simulink model "ieee_6_bus_modified"  (R2015b)
settings: Solver=VariableStepAuto  StartTime=0.0  StopTime=25  RelTol=1e-3
values from neighbouring files (symbols this model uses):
  Cbase = 1/(100*pi*Xbase)    (= 1.34217357979e-05)    [ieee_6_bus.m]
  Lbase = Xbase/(100*pi)    (= 0.754903726073)    [ieee_6_bus.m]
  Ts = 1e-5    (= 1e-05)    [ieee_6_bus.m]
  Xbase = (Vbase^2)/Sbase    (= 237.16)    [ieee_6_bus.m]
libraries: powerlib x193, powerlib_meascontrol x39, simulink x36, powerlib_extras x4, sps_avr x3
(part 4 of 4)

== system ieee_6_bus_modified/GE2.75 - 1/pitch angle controller ==
  wr : Inport
  Constant1 : Constant  Value=1735/1500  SampleTime=Ts
  pitch angle controller : Subsystem
  Beta : Outport
  wires:
  wr/1 -> pitch angle controller/1(wg)
  pitch angle controller/1(pitch) -> Beta/1
  Constant1/1 -> pitch angle controller/2(Ref)

== system ieee_6_bus_modified/GE2.75 - 2/Gearbox ==
  Tt : Inport
  Divide : Product  Inputs=*/
  Gear Ratio1 : Constant  Value=gear
  Tt' : Outport
  wires:
  Gear Ratio1/1 -> Divide/2
  Tt/1 -> Divide/1
  Divide/1 -> Tt'/1

== system ieee_6_bus_modified/GE2.75 - 2/Subsystem ==
  In1 : Inport
  Enable : EnablePort
  Out1 : Outport
  wires:
  In1/1 -> Out1/1

== system ieee_6_bus_modified/GE2.75 - 2/Subsystem1 ==
  In1 : Inport
  Enable : EnablePort
  Out1 : Outport
  wires:
  In1/1 -> Out1/1

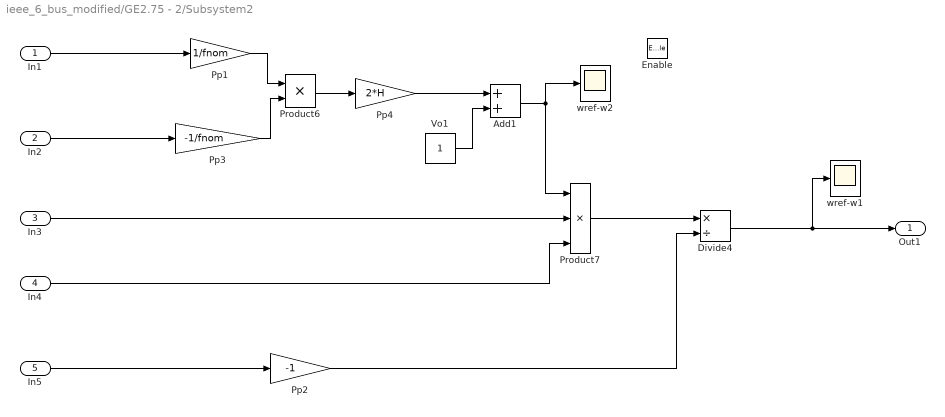
== system ieee_6_bus_modified/GE2.75 - 2/Subsystem2 ==
  In1 : Inport
  In2 : Inport  Port=2
  In3 : Inport  Port=3
  In4 : Inport  Port=4
  In5 : Inport  Port=5
  Enable : EnablePort
  Add1 : Sum
  Divide4 : Product  Inputs=*/
  Pp1 : Gain  Gain=1/fnom
  Pp2 : Gain  Gain=-1
  Pp3 : Gain  Gain=-1/fnom
  Pp4 : Gain  Gain=2*H
  Product6 : Product
  Product7 : Product  Inputs=3
  Vo1 : Constant
  wref-w1 : Scope
  wref-w2 : Scope
  Out1 : Outport
  wires:
  Pp3/1 -> Product6/2
  In2/1 -> Pp3/1
  In3/1 -> Product7/2
  In5/1 -> Pp2/1
  Pp1/1 -> Product6/1
  Vo1/1 -> Add1/2
  Add1/1 -> Product7/1, wref-w2/1
  Product6/1 -> Pp4/1
  Product7/1 -> Divide4/1
  In4/1 -> Product7/3
  Divide4/1 -> wref-w1/1, Out1/1
  In1/1 -> Pp1/1
  Pp4/1 -> Add1/1
  Pp2/1 -> Divide4/2

== system ieee_6_bus_modified/GE2.75 - 2/pitch angle controller ==
  wr : Inport
  Constant1 : Constant  Value=1735/1500  SampleTime=Ts
  pitch angle controller : Subsystem
  Beta : Outport
  wires:
  Constant1/1 -> pitch angle controller/2(Ref)
  pitch angle controller/1(pitch) -> Beta/1
  wr/1 -> pitch angle controller/1(wg)

== system ieee_6_bus_modified/GE2.75 - 3/Gearbox ==
  Tt : Inport
  Divide : Product  Inputs=*/
  Gear Ratio1 : Constant  Value=gear
  Tt' : Outport
  wires:
  Divide/1 -> Tt'/1
  Tt/1 -> Divide/1
  Gear Ratio1/1 -> Divide/2

== system ieee_6_bus_modified/GE2.75 - 3/Subsystem ==
  In1 : Inport
  Enable : EnablePort
  Out1 : Outport
  wires:
  In1/1 -> Out1/1

== system ieee_6_bus_modified/GE2.75 - 3/Subsystem1 ==
  In1 : Inport
  Enable : EnablePort
  Out1 : Outport
  wires:
  In1/1 -> Out1/1

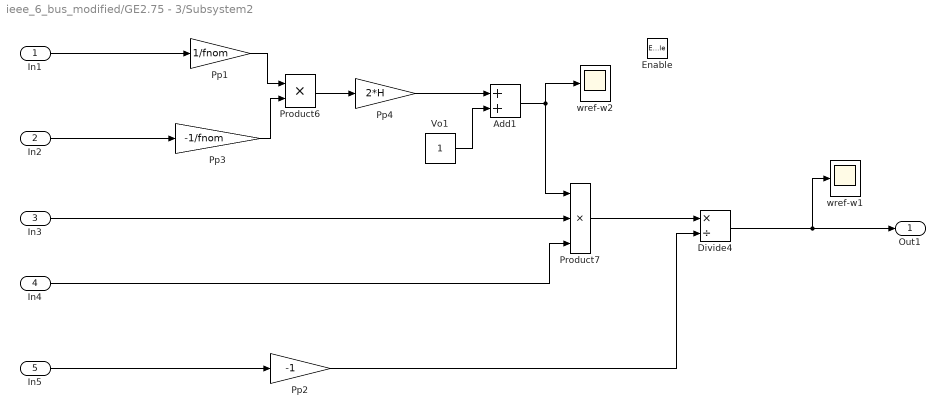
== system ieee_6_bus_modified/GE2.75 - 3/Subsystem2 ==
  In1 : Inport
  In2 : Inport  Port=2
  In3 : Inport  Port=3
  In4 : Inport  Port=4
  In5 : Inport  Port=5
  Enable : EnablePort
  Add1 : Sum
  Divide4 : Product  Inputs=*/
  Pp1 : Gain  Gain=1/fnom
  Pp2 : Gain  Gain=-1
  Pp3 : Gain  Gain=-1/fnom
  Pp4 : Gain  Gain=2*H
  Product6 : Product
  Product7 : Product  Inputs=3
  Vo1 : Constant
  wref-w1 : Scope
  wref-w2 : Scope
  Out1 : Outport
  wires:
  Pp2/1 -> Divide4/2
  Pp4/1 -> Add1/1
  In1/1 -> Pp1/1
  Divide4/1 -> Out1/1, wref-w1/1
  In4/1 -> Product7/3
  Product7/1 -> Divide4/1
  Product6/1 -> Pp4/1
  Add1/1 -> wref-w2/1, Product7/1
  Vo1/1 -> Add1/2
  Pp1/1 -> Product6/1
  In5/1 -> Pp2/1
  In3/1 -> Product7/2
  In2/1 -> Pp3/1
  Pp3/1 -> Product6/2

== system ieee_6_bus_modified/GE2.75 - 3/pitch angle controller ==
  wr : Inport
  Constant1 : Constant  Value=1735/1500  SampleTime=Ts
  pitch angle controller : Subsystem
  Beta : Outport
  wires:
  wr/1 -> pitch angle controller/1(wg)
  pitch angle controller/1(pitch) -> Beta/1
  Constant1/1 -> pitch angle controller/2(Ref)

== system ieee_6_bus_modified/GE2.75 - 4/Gearbox ==
  Tt : Inport
  Divide : Product  Inputs=*/
  Gear Ratio1 : Constant  Value=gear
  Tt' : Outport
  wires:
  Gear Ratio1/1 -> Divide/2
  Tt/1 -> Divide/1
  Divide/1 -> Tt'/1

== system ieee_6_bus_modified/GE2.75 - 4/Subsystem ==
  In1 : Inport
  Enable : EnablePort
  Out1 : Outport
  wires:
  In1/1 -> Out1/1

== system ieee_6_bus_modified/GE2.75 - 4/Subsystem1 ==
  In1 : Inport
  Enable : EnablePort
  Out1 : Outport
  wires:
  In1/1 -> Out1/1

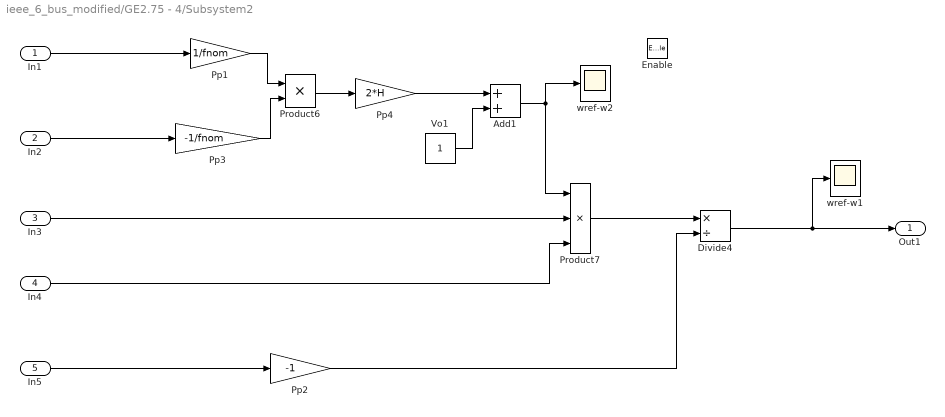
== system ieee_6_bus_modified/GE2.75 - 4/Subsystem2 ==
  In1 : Inport
  In2 : Inport  Port=2
  In3 : Inport  Port=3
  In4 : Inport  Port=4
  In5 : Inport  Port=5
  Enable : EnablePort
  Add1 : Sum
  Divide4 : Product  Inputs=*/
  Pp1 : Gain  Gain=1/fnom
  Pp2 : Gain  Gain=-1
  Pp3 : Gain  Gain=-1/fnom
  Pp4 : Gain  Gain=2*H
  Product6 : Product
  Product7 : Product  Inputs=3
  Vo1 : Constant
  wref-w1 : Scope
  wref-w2 : Scope
  Out1 : Outport
  wires:
  Pp3/1 -> Product6/2
  In2/1 -> Pp3/1
  In3/1 -> Product7/2
  In5/1 -> Pp2/1
  Pp1/1 -> Product6/1
  Vo1/1 -> Add1/2
  Add1/1 -> Product7/1, wref-w2/1
  Product6/1 -> Pp4/1
  Product7/1 -> Divide4/1
  In4/1 -> Product7/3
  Divide4/1 -> wref-w1/1, Out1/1
  In1/1 -> Pp1/1
  Pp4/1 -> Add1/1
  Pp2/1 -> Divide4/2

== system ieee_6_bus_modified/GE2.75 - 4/pitch angle controller ==
  wr : Inport
  Constant1 : Constant  Value=1735/1500  SampleTime=Ts
  pitch angle controller : Subsystem
  Beta : Outport
  wires:
  Constant1/1 -> pitch angle controller/2(Ref)
  pitch angle controller/1(pitch) -> Beta/1
  wr/1 -> pitch angle controller/1(wg)

== system ieee_6_bus_modified/Gen2/B//2 ==
  R2-1 : powerlib/Elements/Series RLC Branch  LConnTagsString=__new0  RConnTagsString=__new0  BranchType=R  Resistance=10000000000  Inductance=1e-3  SetiL0=off  InitialCurrent=0  Capacitance=1000000*Cbase  Setx0=off  InitialVoltage=0  Measurements=None
  R2-2 : powerlib/Elements/Series RLC Branch  LConnTagsString=__new0  RConnTagsString=__new0  BranchType=R  Resistance=10000000000  Inductance=1e-3  SetiL0=off  InitialCurrent=0  Capacitance=1000000*Cbase  Setx0=off  InitialVoltage=0  Measurements=None
  R2-32 : powerlib/Elements/Series RLC Branch  LConnTagsString=__new0  RConnTagsString=__new0  BranchType=R  Resistance=10000000000  Inductance=1e-3  SetiL0=off  InitialCurrent=0  Capacitance=1000000*Cbase  Setx0=off  InitialVoltage=0  Measurements=None
  Conn1 : PMIOPort  Port=1  Side=Right
  Conn2 : PMIOPort  Port=2  Side=Right
  Conn3 : PMIOPort  Port=3  Side=Right
  connections:
  R2-1/LConn1 -- Conn2/RConn1
  R2-1/RConn1 -- R2-32/RConn1 -- R2-2/RConn1
  R2-32/LConn1 -- Conn1/RConn1
  R2-2/LConn1 -- Conn3/RConn1

== system ieee_6_bus_modified/Line 2-4/B//1 ==
  Ground : powerlib/Elements/Ground  LConnTagsString=a
  R2-1 : powerlib/Elements/Series RLC Branch  LConnTagsString=__new0  RConnTagsString=__new0  BranchType=C  Resistance=1  Inductance=1e-3  SetiL0=off  InitialCurrent=0  Capacitance=Cbase/50  Setx0=off  InitialVoltage=0  Measurements=None
  R2-2 : powerlib/Elements/Series RLC Branch  LConnTagsString=__new0  RConnTagsString=__new0  BranchType=C  Resistance=1  Inductance=1e-3  SetiL0=off  InitialCurrent=0  Capacitance=Cbase/50  Setx0=off  InitialVoltage=0  Measurements=None
  R2-32 : powerlib/Elements/Series RLC Branch  LConnTagsString=__new0  RConnTagsString=__new0  BranchType=C  Resistance=1  Inductance=1e-3  SetiL0=off  InitialCurrent=0  Capacitance=Cbase/50  Setx0=off  InitialVoltage=0  Measurements=None
  Conn1 : PMIOPort  Port=1  Side=Right
  Conn2 : PMIOPort  Port=2  Side=Right
  Conn3 : PMIOPort  Port=3  Side=Right
  connections:
  R2-32/LConn1 -- Conn1/RConn1
  R2-2/RConn1 -- R2-32/RConn1 -- Ground/LConn1 -- R2-1/RConn1
  R2-2/LConn1 -- Conn3/RConn1
  R2-1/LConn1 -- Conn2/RConn1

== system ieee_6_bus_modified/Line 2-4/B//2 ==
  Ground : powerlib/Elements/Ground  LConnTagsString=a
  R2-1 : powerlib/Elements/Series RLC Branch  LConnTagsString=__new0  RConnTagsString=__new0  BranchType=C  Resistance=1  Inductance=1e-3  SetiL0=off  InitialCurrent=0  Capacitance=Cbase/50  Setx0=off  InitialVoltage=0  Measurements=None
  R2-2 : powerlib/Elements/Series RLC Branch  LConnTagsString=__new0  RConnTagsString=__new0  BranchType=C  Resistance=1  Inductance=1e-3  SetiL0=off  InitialCurrent=0  Capacitance=Cbase/50  Setx0=off  InitialVoltage=0  Measurements=None
  R2-32 : powerlib/Elements/Series RLC Branch  LConnTagsString=__new0  RConnTagsString=__new0  BranchType=C  Resistance=1  Inductance=1e-3  SetiL0=off  InitialCurrent=0  Capacitance=Cbase/50  Setx0=off  InitialVoltage=0  Measurements=None
  Conn1 : PMIOPort  Port=1  Side=Right
  Conn2 : PMIOPort  Port=2  Side=Right
  Conn3 : PMIOPort  Port=3  Side=Right
  connections:
  R2-1/LConn1 -- Conn2/RConn1
  R2-2/LConn1 -- Conn3/RConn1
  Ground/LConn1 -- R2-2/RConn1 -- R2-1/RConn1 -- R2-32/RConn1
  R2-32/LConn1 -- Conn1/RConn1

== system ieee_6_bus_modified/Subsystem/B//1 ==
  C1 : powerlib/Elements/Series RLC Branch  LConnTagsString=__new0  RConnTagsString=__new0  BranchType=C  Resistance=1  Inductance=1e-3  SetiL0=off  InitialCurrent=0  Capacitance=Cbase/25  Setx0=off  InitialVoltage=0  Measurements=None
  C2 : powerlib/Elements/Series RLC Branch  LConnTagsString=__new0  RConnTagsString=__new0  BranchType=C  Resistance=1  Inductance=1e-3  SetiL0=off  InitialCurrent=0  Capacitance=Cbase/25  Setx0=off  InitialVoltage=0  Measurements=None
  C3 : powerlib/Elements/Series RLC Branch  LConnTagsString=__new0  RConnTagsString=__new0  BranchType=C  Resistance=1  Inductance=1e-3  SetiL0=off  InitialCurrent=0  Capacitance=Cbase/25  Setx0=off  InitialVoltage=0  Measurements=None
  Ground : powerlib/Elements/Ground  LConnTagsString=a
  Conn1 : PMIOPort  Port=1  Side=Right
  Conn2 : PMIOPort  Port=2  Side=Right
  Conn3 : PMIOPort  Port=3  Side=Right
  connections:
  C1/LConn1 -- Conn1/RConn1
  C3/RConn1 -- Ground/LConn1 -- C1/RConn1 -- C2/RConn1
  C3/LConn1 -- Conn3/RConn1
  C2/LConn1 -- Conn2/RConn1

== system ieee_6_bus_modified/Subsystem/B//3 ==
  C1 : powerlib/Elements/Series RLC Branch  LConnTagsString=__new0  RConnTagsString=__new0  BranchType=C  Resistance=1  Inductance=1e-3  SetiL0=off  InitialCurrent=0  Capacitance=Cbase/25  Setx0=off  InitialVoltage=0  Measurements=None
  C2 : powerlib/Elements/Series RLC Branch  LConnTagsString=__new0  RConnTagsString=__new0  BranchType=C  Resistance=1  Inductance=1e-3  SetiL0=off  InitialCurrent=0  Capacitance=Cbase/25  Setx0=off  InitialVoltage=0  Measurements=None
  C3 : powerlib/Elements/Series RLC Branch  LConnTagsString=__new0  RConnTagsString=__new0  BranchType=C  Resistance=1  Inductance=1e-3  SetiL0=off  InitialCurrent=0  Capacitance=Cbase/25  Setx0=off  InitialVoltage=0  Measurements=None
  Ground : powerlib/Elements/Ground  LConnTagsString=a
  Conn1 : PMIOPort  Port=1  Side=Right
  Conn2 : PMIOPort  Port=2  Side=Right
  Conn3 : PMIOPort  Port=3  Side=Right
  connections:
  C2/LConn1 -- Conn2/RConn1
  C3/LConn1 -- Conn3/RConn1
  C1/RConn1 -- C3/RConn1 -- C2/RConn1 -- Ground/LConn1
  C1/LConn1 -- Conn1/RConn1

== system ieee_6_bus_modified/Subsystem1/B//1 ==
  Ground : powerlib/Elements/Ground  LConnTagsString=a
  R2-1 : powerlib/Elements/Series RLC Branch  LConnTagsString=__new0  RConnTagsString=__new0  BranchType=C  Resistance=1  Inductance=1e-3  SetiL0=off  InitialCurrent=0  Capacitance=Cbase/25  Setx0=off  InitialVoltage=0  Measurements=None
  R2-2 : powerlib/Elements/Series RLC Branch  LConnTagsString=__new0  RConnTagsString=__new0  BranchType=C  Resistance=1  Inductance=1e-3  SetiL0=off  InitialCurrent=0  Capacitance=Cbase/25  Setx0=off  InitialVoltage=0  Measurements=None
  R2-32 : powerlib/Elements/Series RLC Branch  LConnTagsString=__new0  RConnTagsString=__new0  BranchType=C  Resistance=1  Inductance=1e-3  SetiL0=off  InitialCurrent=0  Capacitance=Cbase/25  Setx0=off  InitialVoltage=0  Measurements=None
  Conn1 : PMIOPort  Port=1  Side=Right
  Conn2 : PMIOPort  Port=2  Side=Right
  Conn3 : PMIOPort  Port=3  Side=Right
  connections:
  R2-32/LConn1 -- Conn1/RConn1
  R2-2/RConn1 -- Ground/LConn1 -- R2-32/RConn1 -- R2-1/RConn1
  R2-2/LConn1 -- Conn3/RConn1
  R2-1/LConn1 -- Conn2/RConn1

== system ieee_6_bus_modified/Subsystem1/B//5 ==
  Ground : powerlib/Elements/Ground  LConnTagsString=a
  R2-1 : powerlib/Elements/Series RLC Branch  LConnTagsString=__new0  RConnTagsString=__new0  BranchType=C  Resistance=1  Inductance=1e-3  SetiL0=off  InitialCurrent=0  Capacitance=Cbase/25  Setx0=off  InitialVoltage=0  Measurements=None
  R2-2 : powerlib/Elements/Series RLC Branch  LConnTagsString=__new0  RConnTagsString=__new0  BranchType=C  Resistance=1  Inductance=1e-3  SetiL0=off  InitialCurrent=0  Capacitance=Cbase/25  Setx0=off  InitialVoltage=0  Measurements=None
  R2-32 : powerlib/Elements/Series RLC Branch  LConnTagsString=__new0  RConnTagsString=__new0  BranchType=C  Resistance=1  Inductance=1e-3  SetiL0=off  InitialCurrent=0  Capacitance=Cbase/25  Setx0=off  InitialVoltage=0  Measurements=None
  Conn1 : PMIOPort  Port=1  Side=Right
  Conn2 : PMIOPort  Port=2  Side=Right
  Conn3 : PMIOPort  Port=3  Side=Right
  connections:
  R2-1/LConn1 -- Conn2/RConn1
  R2-2/LConn1 -- Conn3/RConn1
  R2-32/RConn1 -- R2-2/RConn1 -- R2-1/RConn1 -- Ground/LConn1
  R2-32/LConn1 -- Conn1/RConn1

== system ieee_6_bus_modified/Subsystem2/B//7 ==
  Ground : powerlib/Elements/Ground  LConnTagsString=a
  R2-1 : powerlib/Elements/Series RLC Branch  LConnTagsString=__new0  RConnTagsString=__new0  BranchType=C  Resistance=1  Inductance=1e-3  SetiL0=off  InitialCurrent=0  Capacitance=Cbase/12.5  Setx0=off  InitialVoltage=0  Measurements=None
  R2-2 : powerlib/Elements/Series RLC Branch  LConnTagsString=__new0  RConnTagsString=__new0  BranchType=C  Resistance=1  Inductance=1e-3  SetiL0=off  InitialCurrent=0  Capacitance=Cbase/12.5  Setx0=off  InitialVoltage=0  Measurements=None
  R2-32 : powerlib/Elements/Series RLC Branch  LConnTagsString=__new0  RConnTagsString=__new0  BranchType=C  Resistance=1  Inductance=1e-3  SetiL0=off  InitialCurrent=0  Capacitance=Cbase/12.5  Setx0=off  InitialVoltage=0  Measurements=None
  Conn1 : PMIOPort  Port=1  Side=Right
  Conn2 : PMIOPort  Port=2  Side=Right
  Conn3 : PMIOPort  Port=3  Side=Right
  connections:
  R2-1/LConn1 -- Conn2/RConn1
  R2-2/LConn1 -- Conn3/RConn1
  R2-2/RConn1 -- R2-32/RConn1 -- Ground/LConn1 -- R2-1/RConn1
  R2-32/LConn1 -- Conn1/RConn1

== system ieee_6_bus_modified/Subsystem2/B//8 ==
  Ground : powerlib/Elements/Ground  LConnTagsString=a
  R2-1 : powerlib/Elements/Series RLC Branch  LConnTagsString=__new0  RConnTagsString=__new0  BranchType=C  Resistance=1  Inductance=1e-3  SetiL0=off  InitialCurrent=0  Capacitance=Cbase/12.5  Setx0=off  InitialVoltage=0  Measurements=None
  R2-2 : powerlib/Elements/Series RLC Branch  LConnTagsString=__new0  RConnTagsString=__new0  BranchType=C  Resistance=1  Inductance=1e-3  SetiL0=off  InitialCurrent=0  Capacitance=Cbase/12.5  Setx0=off  InitialVoltage=0  Measurements=None
  R2-32 : powerlib/Elements/Series RLC Branch  LConnTagsString=__new0  RConnTagsString=__new0  BranchType=C  Resistance=1  Inductance=1e-3  SetiL0=off  InitialCurrent=0  Capacitance=Cbase/12.5  Setx0=off  InitialVoltage=0  Measurements=None
  Conn1 : PMIOPort  Port=1  Side=Right
  Conn2 : PMIOPort  Port=2  Side=Right
  Conn3 : PMIOPort  Port=3  Side=Right
  connections:
  R2-32/LConn1 -- Conn1/RConn1
  Ground/LConn1 -- R2-2/RConn1 -- R2-1/RConn1 -- R2-32/RConn1
  R2-2/LConn1 -- Conn3/RConn1
  R2-1/LConn1 -- Conn2/RConn1

== system ieee_6_bus_modified/Subsystem3/B//11 ==
  Ground : powerlib/Elements/Ground  LConnTagsString=a
  R2-1 : powerlib/Elements/Series RLC Branch  LConnTagsString=__new0  RConnTagsString=__new0  BranchType=C  Resistance=1  Inductance=1e-3  SetiL0=off  InitialCurrent=0  Capacitance=(6*Cbase)/100  Setx0=off  InitialVoltage=0  Measurements=None
  R2-2 : powerlib/Elements/Series RLC Branch  LConnTagsString=__new0  RConnTagsString=__new0  BranchType=C  Resistance=1  Inductance=1e-3  SetiL0=off  InitialCurrent=0  Capacitance=(6*Cbase)/100  Setx0=off  InitialVoltage=0  Measurements=None
  R2-32 : powerlib/Elements/Series RLC Branch  LConnTagsString=__new0  RConnTagsString=__new0  BranchType=C  Resistance=1  Inductance=1e-3  SetiL0=off  InitialCurrent=0  Capacitance=(6*Cbase)/100  Setx0=off  InitialVoltage=0  Measurements=None
  Conn1 : PMIOPort  Port=1  Side=Right
  Conn2 : PMIOPort  Port=2  Side=Right
  Conn3 : PMIOPort  Port=3  Side=Right
  connections:
  R2-1/LConn1 -- Conn2/RConn1
  R2-2/LConn1 -- Conn3/RConn1
  R2-32/RConn1 -- R2-2/RConn1 -- R2-1/RConn1 -- Ground/LConn1
  R2-32/LConn1 -- Conn1/RConn1

== system ieee_6_bus_modified/Subsystem3/B//12 ==
  Ground : powerlib/Elements/Ground  LConnTagsString=a
  R2-1 : powerlib/Elements/Series RLC Branch  LConnTagsString=__new0  RConnTagsString=__new0  BranchType=C  Resistance=1  Inductance=1e-3  SetiL0=off  InitialCurrent=0  Capacitance=(6*Cbase)/100  Setx0=off  InitialVoltage=0  Measurements=None
  R2-2 : powerlib/Elements/Series RLC Branch  LConnTagsString=__new0  RConnTagsString=__new0  BranchType=C  Resistance=1  Inductance=1e-3  SetiL0=off  InitialCurrent=0  Capacitance=(6*Cbase)/100  Setx0=off  InitialVoltage=0  Measurements=None
  R2-32 : powerlib/Elements/Series RLC Branch  LConnTagsString=__new0  RConnTagsString=__new0  BranchType=C  Resistance=1  Inductance=1e-3  SetiL0=off  InitialCurrent=0  Capacitance=(6*Cbase)/100  Setx0=off  InitialVoltage=0  Measurements=None
  Conn1 : PMIOPort  Port=1  Side=Right
  Conn2 : PMIOPort  Port=2  Side=Right
  Conn3 : PMIOPort  Port=3  Side=Right
  connections:
  R2-32/LConn1 -- Conn1/RConn1
  R2-2/RConn1 -- Ground/LConn1 -- R2-32/RConn1 -- R2-1/RConn1
  R2-2/LConn1 -- Conn3/RConn1
  R2-1/LConn1 -- Conn2/RConn1

== system ieee_6_bus_modified/Subsystem4/B//19 ==
  Ground : powerlib/Elements/Ground  LConnTagsString=a
  R2-1 : powerlib/Elements/Series RLC Branch  LConnTagsString=__new0  RConnTagsString=__new0  BranchType=C  Resistance=1  Inductance=1e-3  SetiL0=off  InitialCurrent=0  Capacitance=Cbase/20  Setx0=off  InitialVoltage=0  Measurements=None
  R2-2 : powerlib/Elements/Series RLC Branch  LConnTagsString=__new0  RConnTagsString=__new0  BranchType=C  Resistance=1  Inductance=1e-3  SetiL0=off  InitialCurrent=0  Capacitance=Cbase/20  Setx0=off  InitialVoltage=0  Measurements=None
  R2-32 : powerlib/Elements/Series RLC Branch  LConnTagsString=__new0  RConnTagsString=__new0  BranchType=C  Resistance=1  Inductance=1e-3  SetiL0=off  InitialCurrent=0  Capacitance=Cbase/20  Setx0=off  InitialVoltage=0  Measurements=None
  Conn1 : PMIOPort  Port=1  Side=Right
  Conn2 : PMIOPort  Port=2  Side=Right
  Conn3 : PMIOPort  Port=3  Side=Right
  connections:
  R2-1/LConn1 -- Conn2/RConn1
  R2-2/LConn1 -- Conn3/RConn1
  R2-32/RConn1 -- R2-2/RConn1 -- R2-1/RConn1 -- Ground/LConn1
  R2-32/LConn1 -- Conn1/RConn1

== system ieee_6_bus_modified/Subsystem4/B//20 ==
  Ground : powerlib/Elements/Ground  LConnTagsString=a
  R2-1 : powerlib/Elements/Series RLC Branch  LConnTagsString=__new0  RConnTagsString=__new0  BranchType=C  Resistance=1  Inductance=1e-3  SetiL0=off  InitialCurrent=0  Capacitance=Cbase/20  Setx0=off  InitialVoltage=0  Measurements=None
  R2-2 : powerlib/Elements/Series RLC Branch  LConnTagsString=__new0  RConnTagsString=__new0  BranchType=C  Resistance=1  Inductance=1e-3  SetiL0=off  InitialCurrent=0  Capacitance=Cbase/20  Setx0=off  InitialVoltage=0  Measurements=None
  R2-32 : powerlib/Elements/Series RLC Branch  LConnTagsString=__new0  RConnTagsString=__new0  BranchType=C  Resistance=1  Inductance=1e-3  SetiL0=off  InitialCurrent=0  Capacitance=Cbase/20  Setx0=off  InitialVoltage=0  Measurements=None
  Conn1 : PMIOPort  Port=1  Side=Right
  Conn2 : PMIOPort  Port=2  Side=Right
  Conn3 : PMIOPort  Port=3  Side=Right
  connections:
  R2-32/LConn1 -- Conn1/RConn1
  R2-2/RConn1 -- Ground/LConn1 -- R2-32/RConn1 -- R2-1/RConn1
  R2-2/LConn1 -- Conn3/RConn1
  R2-1/LConn1 -- Conn2/RConn1

== system ieee_6_bus_modified/Subsystem5/B//10 ==
  Ground : powerlib/Elements/Ground  LConnTagsString=a
  R2-1 : powerlib/Elements/Series RLC Branch  LConnTagsString=__new0  RConnTagsString=__new0  BranchType=C  Resistance=1  Inductance=1e-3  SetiL0=off  InitialCurrent=0  Capacitance=Cbase/50  Setx0=off  InitialVoltage=0  Measurements=None
  R2-2 : powerlib/Elements/Series RLC Branch  LConnTagsString=__new0  RConnTagsString=__new0  BranchType=C  Resistance=1  Inductance=1e-3  SetiL0=off  InitialCurrent=0  Capacitance=Cbase/50  Setx0=off  InitialVoltage=0  Measurements=None
  R2-32 : powerlib/Elements/Series RLC Branch  LConnTagsString=__new0  RConnTagsString=__new0  BranchType=C  Resistance=1  Inductance=1e-3  SetiL0=off  InitialCurrent=0  Capacitance=Cbase/50  Setx0=off  InitialVoltage=0  Measurements=None
  Conn1 : PMIOPort  Port=1  Side=Right
  Conn2 : PMIOPort  Port=2  Side=Right
  Conn3 : PMIOPort  Port=3  Side=Right
  connections:
  R2-1/LConn1 -- Conn2/RConn1
  R2-2/LConn1 -- Conn3/RConn1
  R2-2/RConn1 -- R2-32/RConn1 -- Ground/LConn1 -- R2-1/RConn1
  R2-32/LConn1 -- Conn1/RConn1

== system ieee_6_bus_modified/Subsystem5/B//9 ==
  Ground : powerlib/Elements/Ground  LConnTagsString=a
  R2-1 : powerlib/Elements/Series RLC Branch  LConnTagsString=__new0  RConnTagsString=__new0  BranchType=C  Resistance=1  Inductance=1e-3  SetiL0=off  InitialCurrent=0  Capacitance=Cbase/50  Setx0=off  InitialVoltage=0  Measurements=None
  R2-2 : powerlib/Elements/Series RLC Branch  LConnTagsString=__new0  RConnTagsString=__new0  BranchType=C  Resistance=1  Inductance=1e-3  SetiL0=off  InitialCurrent=0  Capacitance=Cbase/50  Setx0=off  InitialVoltage=0  Measurements=None
  R2-32 : powerlib/Elements/Series RLC Branch  LConnTagsString=__new0  RConnTagsString=__new0  BranchType=C  Resistance=1  Inductance=1e-3  SetiL0=off  InitialCurrent=0  Capacitance=Cbase/50  Setx0=off  InitialVoltage=0  Measurements=None
  Conn1 : PMIOPort  Port=1  Side=Right
  Conn2 : PMIOPort  Port=2  Side=Right
  Conn3 : PMIOPort  Port=3  Side=Right
  connections:
  R2-32/LConn1 -- Conn1/RConn1
  Ground/LConn1 -- R2-2/RConn1 -- R2-1/RConn1 -- R2-32/RConn1
  R2-2/LConn1 -- Conn3/RConn1
  R2-1/LConn1 -- Conn2/RConn1

== system ieee_6_bus_modified/Subsystem6/B//16 ==
  C1 : powerlib/Elements/Series RLC Branch  LConnTagsString=__new0  RConnTagsString=__new0  BranchType=C  Resistance=1  Inductance=1e-3  SetiL0=off  InitialCurrent=0  Capacitance=Cbase/25  Setx0=off  InitialVoltage=0  Measurements=None
  C2 : powerlib/Elements/Series RLC Branch  LConnTagsString=__new0  RConnTagsString=__new0  BranchType=C  Resistance=1  Inductance=1e-3  SetiL0=off  InitialCurrent=0  Capacitance=Cbase/25  Setx0=off  InitialVoltage=0  Measurements=None
  C3 : powerlib/Elements/Series RLC Branch  LConnTagsString=__new0  RConnTagsString=__new0  BranchType=C  Resistance=1  Inductance=1e-3  SetiL0=off  InitialCurrent=0  Capacitance=Cbase/25  Setx0=off  InitialVoltage=0  Measurements=None
  Ground : powerlib/Elements/Ground  LConnTagsString=a
  Conn1 : PMIOPort  Port=1  Side=Right
  Conn2 : PMIOPort  Port=2  Side=Right
  Conn3 : PMIOPort  Port=3  Side=Right
  connections:
  C1/LConn1 -- Conn1/RConn1
  Ground/LConn1 -- C3/RConn1 -- C2/RConn1 -- C1/RConn1
  C3/LConn1 -- Conn3/RConn1
  C2/LConn1 -- Conn2/RConn1

== system ieee_6_bus_modified/Subsystem6/B//18 ==
  C1 : powerlib/Elements/Series RLC Branch  LConnTagsString=__new0  RConnTagsString=__new0  BranchType=C  Resistance=1  Inductance=1e-3  SetiL0=off  InitialCurrent=0  Capacitance=Cbase/25  Setx0=off  InitialVoltage=0  Measurements=None
  C2 : powerlib/Elements/Series RLC Branch  LConnTagsString=__new0  RConnTagsString=__new0  BranchType=C  Resistance=1  Inductance=1e-3  SetiL0=off  InitialCurrent=0  Capacitance=Cbase/25  Setx0=off  InitialVoltage=0  Measurements=None
  C3 : powerlib/Elements/Series RLC Branch  LConnTagsString=__new0  RConnTagsString=__new0  BranchType=C  Resistance=1  Inductance=1e-3  SetiL0=off  InitialCurrent=0  Capacitance=Cbase/25  Setx0=off  InitialVoltage=0  Measurements=None
  Ground : powerlib/Elements/Ground  LConnTagsString=a
  Conn1 : PMIOPort  Port=1  Side=Right
  Conn2 : PMIOPort  Port=2  Side=Right
  Conn3 : PMIOPort  Port=3  Side=Right
  connections:
  C2/LConn1 -- Conn2/RConn1
  C3/LConn1 -- Conn3/RConn1
  C3/RConn1 -- C1/RConn1 -- Ground/LConn1 -- C2/RConn1
  C1/LConn1 -- Conn1/RConn1

== system ieee_6_bus_modified/Subsystem7/B//13 ==
  Ground : powerlib/Elements/Ground  LConnTagsString=a
  R2-1 : powerlib/Elements/Series RLC Branch  LConnTagsString=__new0  RConnTagsString=__new0  BranchType=C  Resistance=1  Inductance=1e-3  SetiL0=off  InitialCurrent=0  Capacitance=Cbase/20  Setx0=off  InitialVoltage=0  Measurements=None
  R2-2 : powerlib/Elements/Series RLC Branch  LConnTagsString=__new0  RConnTagsString=__new0  BranchType=C  Resistance=1  Inductance=1e-3  SetiL0=off  InitialCurrent=0  Capacitance=Cbase/20  Setx0=off  InitialVoltage=0  Measurements=None
  R2-32 : powerlib/Elements/Series RLC Branch  LConnTagsString=__new0  RConnTagsString=__new0  BranchType=C  Resistance=1  Inductance=1e-3  SetiL0=off  InitialCurrent=0  Capacitance=Cbase/20  Setx0=off  InitialVoltage=0  Measurements=None
  Conn1 : PMIOPort  Port=1  Side=Right
  Conn2 : PMIOPort  Port=2  Side=Right
  Conn3 : PMIOPort  Port=3  Side=Right
  connections:
  R2-1/LConn1 -- Conn2/RConn1
  R2-2/LConn1 -- Conn3/RConn1
  R2-2/RConn1 -- R2-32/RConn1 -- Ground/LConn1 -- R2-1/RConn1
  R2-32/LConn1 -- Conn1/RConn1

== system ieee_6_bus_modified/Subsystem7/B//14 ==
  Ground : powerlib/Elements/Ground  LConnTagsString=a
  R2-1 : powerlib/Elements/Series RLC Branch  LConnTagsString=__new0  RConnTagsString=__new0  BranchType=C  Resistance=1  Inductance=1e-3  SetiL0=off  InitialCurrent=0  Capacitance=Cbase/20  Setx0=off  InitialVoltage=0  Measurements=None
  R2-2 : powerlib/Elements/Series RLC Branch  LConnTagsString=__new0  RConnTagsString=__new0  BranchType=C  Resistance=1  Inductance=1e-3  SetiL0=off  InitialCurrent=0  Capacitance=Cbase/20  Setx0=off  InitialVoltage=0  Measurements=None
  R2-32 : powerlib/Elements/Series RLC Branch  LConnTagsString=__new0  RConnTagsString=__new0  BranchType=C  Resistance=1  Inductance=1e-3  SetiL0=off  InitialCurrent=0  Capacitance=Cbase/20  Setx0=off  InitialVoltage=0  Measurements=None
  Conn1 : PMIOPort  Port=1  Side=Right
  Conn2 : PMIOPort  Port=2  Side=Right
  Conn3 : PMIOPort  Port=3  Side=Right
  connections:
  R2-32/LConn1 -- Conn1/RConn1
  Ground/LConn1 -- R2-2/RConn1 -- R2-1/RConn1 -- R2-32/RConn1
  R2-2/LConn1 -- Conn3/RConn1
  R2-1/LConn1 -- Conn2/RConn1

== system ieee_6_bus_modified/Subsystem8/B//21 ==
  C1 : powerlib/Elements/Series RLC Branch  LConnTagsString=__new0  RConnTagsString=__new0  BranchType=C  Resistance=1  Inductance=1e-3  SetiL0=off  InitialCurrent=0  Capacitance=(6*Cbase)/100  Setx0=off  InitialVoltage=0  Measurements=None
  C2 : powerlib/Elements/Series RLC Branch  LConnTagsString=__new0  RConnTagsString=__new0  BranchType=C  Resistance=1  Inductance=1e-3  SetiL0=off  InitialCurrent=0  Capacitance=(6*Cbase)/100  Setx0=off  InitialVoltage=0  Measurements=None
  C3 : powerlib/Elements/Series RLC Branch  LConnTagsString=__new0  RConnTagsString=__new0  BranchType=C  Resistance=1  Inductance=1e-3  SetiL0=off  InitialCurrent=0  Capacitance=(6*Cbase)/100  Setx0=off  InitialVoltage=0  Measurements=None
  Ground : powerlib/Elements/Ground  LConnTagsString=a
  Conn1 : PMIOPort  Port=1  Side=Right
  Conn2 : PMIOPort  Port=2  Side=Right
  Conn3 : PMIOPort  Port=3  Side=Right
  connections:
  C2/LConn1 -- Conn2/RConn1
  C3/LConn1 -- Conn3/RConn1
  C1/RConn1 -- C3/RConn1 -- C2/RConn1 -- Ground/LConn1
  C1/LConn1 -- Conn1/RConn1

== system ieee_6_bus_modified/Subsystem8/B//22 ==
  C1 : powerlib/Elements/Series RLC Branch  LConnTagsString=__new0  RConnTagsString=__new0  BranchType=C  Resistance=1  Inductance=1e-3  SetiL0=off  InitialCurrent=0  Capacitance=(6*Cbase)/100  Setx0=off  InitialVoltage=0  Measurements=None
  C2 : powerlib/Elements/Series RLC Branch  LConnTagsString=__new0  RConnTagsString=__new0  BranchType=C  Resistance=1  Inductance=1e-3  SetiL0=off  InitialCurrent=0  Capacitance=(6*Cbase)/100  Setx0=off  InitialVoltage=0  Measurements=None
  C3 : powerlib/Elements/Series RLC Branch  LConnTagsString=__new0  RConnTagsString=__new0  BranchType=C  Resistance=1  Inductance=1e-3  SetiL0=off  InitialCurrent=0  Capacitance=(6*Cbase)/100  Setx0=off  InitialVoltage=0  Measurements=None
  Ground : powerlib/Elements/Ground  LConnTagsString=a
  Conn1 : PMIOPort  Port=1  Side=Right
  Conn2 : PMIOPort  Port=2  Side=Right
  Conn3 : PMIOPort  Port=3  Side=Right
  connections:
  C1/LConn1 -- Conn1/RConn1
  C3/RConn1 -- Ground/LConn1 -- C1/RConn1 -- C2/RConn1
  C3/LConn1 -- Conn3/RConn1
  C2/LConn1 -- Conn2/RConn1

== system ieee_6_bus_modified/Subsystem9/B//15 ==
  Ground : powerlib/Elements/Ground  LConnTagsString=a
  R2-1 : powerlib/Elements/Series RLC Branch  LConnTagsString=__new0  RConnTagsString=__new0  BranchType=C  Resistance=1  Inductance=1e-3  SetiL0=off  InitialCurrent=0  Capacitance=(6*Cbase)/100  Setx0=off  InitialVoltage=0  Measurements=None
  R2-2 : powerlib/Elements/Series RLC Branch  LConnTagsString=__new0  RConnTagsString=__new0  BranchType=C  Resistance=1  Inductance=1e-3  SetiL0=off  InitialCurrent=0  Capacitance=(6*Cbase)/100  Setx0=off  InitialVoltage=0  Measurements=None
  R2-32 : powerlib/Elements/Series RLC Branch  LConnTagsString=__new0  RConnTagsString=__new0  BranchType=C  Resistance=1  Inductance=1e-3  SetiL0=off  InitialCurrent=0  Capacitance=(6*Cbase)/100  Setx0=off  InitialVoltage=0  Measurements=None
  Conn1 : PMIOPort  Port=1  Side=Right
  Conn2 : PMIOPort  Port=2  Side=Right
  Conn3 : PMIOPort  Port=3  Side=Right
  connections:
  R2-1/LConn1 -- Conn2/RConn1
  R2-2/LConn1 -- Conn3/RConn1
  R2-32/RConn1 -- R2-2/RConn1 -- R2-1/RConn1 -- Ground/LConn1
  R2-32/LConn1 -- Conn1/RConn1

== system ieee_6_bus_modified/Subsystem9/B//6 ==
  Ground : powerlib/Elements/Ground  LConnTagsString=a
  R2-1 : powerlib/Elements/Series RLC Branch  LConnTagsString=__new0  RConnTagsString=__new0  BranchType=C  Resistance=1  Inductance=1e-3  SetiL0=off  InitialCurrent=0  Capacitance=(6*Cbase)/100  Setx0=off  InitialVoltage=0  Measurements=None
  R2-2 : powerlib/Elements/Series RLC Branch  LConnTagsString=__new0  RConnTagsString=__new0  BranchType=C  Resistance=1  Inductance=1e-3  SetiL0=off  InitialCurrent=0  Capacitance=(6*Cbase)/100  Setx0=off  InitialVoltage=0  Measurements=None
  R2-32 : powerlib/Elements/Series RLC Branch  LConnTagsString=__new0  RConnTagsString=__new0  BranchType=C  Resistance=1  Inductance=1e-3  SetiL0=off  InitialCurrent=0  Capacitance=(6*Cbase)/100  Setx0=off  InitialVoltage=0  Measurements=None
  Conn1 : PMIOPort  Port=1  Side=Right
  Conn2 : PMIOPort  Port=2  Side=Right
  Conn3 : PMIOPort  Port=3  Side=Right
  connections:
  R2-32/LConn1 -- Conn1/RConn1
  R2-2/RConn1 -- Ground/LConn1 -- R2-32/RConn1 -- R2-1/RConn1
  R2-2/LConn1 -- Conn3/RConn1
  R2-1/LConn1 -- Conn2/RConn1

== system ieee_6_bus_modified/GE2.75 - 1/pitch angle controller/pitch angle controller ==
  wg : Inport
  Ref : Inport  Port=2
  "0-pitch_max " : Saturate  UpperLimit=27  LowerLimit=0  SampleTime=Ts
  Discrete PID Controller : simulink/Continuous/PID Controller  Controller=PI  TimeDomain=Discrete-time  SampleTime=Ts  IntegratorMethod=Forward Euler  FilterMethod=Forward Euler  Form=Parallel  UseFilter=on  ControllerParametersSource=internal  P=200  I=25  D=0  N=100  InitialConditionSource=internal  InitialConditionForIntegrator=0  InitialConditionForFilter=0  ExternalReset=none  ZeroCross=off  LimitOutput=on  UpperSaturationLimit=27  LowerSaturationLimit=0  LinearizeAsGain=off  AntiWindupMode=clamping  Kb=1  TrackingMode=off  Kt=1  PParamMin=[]  PParamMax=[]  IParamMin=[]  IParamMax=[]  DParamMin=[]  DParamMax=[]  NParamMin=[]  NParamMax=[]  KbParamMin=[]  KbParamMax=[]  KtParamMin=[]  KtParamMax=[]  POutMin=[]  POutMax=[]  IOutMin=[]  IOutMax=[]  DOutMin=[]  DOutMax=[]  NOutMin=[]  NOutMax=[]  KbOutMin=[]  KbOutMax=[]  KtOutMin=[]  KtOutMax=[]  IntegratorOutMin=[]  IntegratorOutMax=[]  FilterOutMin=[]  FilterOutMax=[]  SumOutMin=[]  SumOutMax=[]  SumI1OutMin=[]  SumI1OutMax=[]  SumI2OutMin=[]  SumI2OutMax=[]  SumI3OutMin=[]  SumI3OutMax=[]  SumDOutMin=[]  SumDOutMax=[]  SaturationOutMin=[]  SaturationOutMax=[]  IntegratorContinuousStateAttributes=''  IntegratorStateMustResolveToSignalObject=off  IntegratorRTWStateStorageClass=Auto  FilterContinuousStateAttributes=''  FilterStateMustResolveToSignalObject=off  FilterRTWStateStorageClass=Auto  DifferentiatorICPrevScaledInput=0  DifferentiatorOutMin=[]  DifferentiatorOutMax=[]
  Rate Limiter : RateLimiter  RisingSlewLimit=10  FallingSlewLimit=-10
  Sum3 : Sum  Inputs=|+-  SampleTime=Ts
  t=Pitch_time_constant1 : powerlib_extras/Discrete  Control Blocks/Discrete 1st-Order Filter  FilterType=Lowpass  Tc=0.02  Ts=Ts  Initialize=on  Vac_Init=[0.8 -25 60]*0  Vdc_Init=0  PlotResponse=off  param1=[1 500 0.1]
  pitch : Outport
  wires:
  Discrete PID Controller/1 -> Rate Limiter/1
  t=Pitch_time_constant1/1 -> pitch/1
  "0-pitch_max "/1 -> t=Pitch_time_constant1/1
  Rate Limiter/1 -> "0-pitch_max "/1
  Ref/1 -> Sum3/2
  wg/1 -> Sum3/1
  Sum3/1 -> Discrete PID Controller/1

== system ieee_6_bus_modified/GE2.75 - 2/pitch angle controller/pitch angle controller ==
  wg : Inport
  Ref : Inport  Port=2
  "0-pitch_max " : Saturate  UpperLimit=27  LowerLimit=0  SampleTime=Ts
  Discrete PID Controller : simulink/Continuous/PID Controller  Controller=PI  TimeDomain=Discrete-time  SampleTime=Ts  IntegratorMethod=Forward Euler  FilterMethod=Forward Euler  Form=Parallel  UseFilter=on  ControllerParametersSource=internal  P=200  I=25  D=0  N=100  InitialConditionSource=internal  InitialConditionForIntegrator=0  InitialConditionForFilter=0  ExternalReset=none  ZeroCross=off  LimitOutput=on  UpperSaturationLimit=27  LowerSaturationLimit=0  LinearizeAsGain=off  AntiWindupMode=clamping  Kb=1  TrackingMode=off  Kt=1  PParamMin=[]  PParamMax=[]  IParamMin=[]  IParamMax=[]  DParamMin=[]  DParamMax=[]  NParamMin=[]  NParamMax=[]  KbParamMin=[]  KbParamMax=[]  KtParamMin=[]  KtParamMax=[]  POutMin=[]  POutMax=[]  IOutMin=[]  IOutMax=[]  DOutMin=[]  DOutMax=[]  NOutMin=[]  NOutMax=[]  KbOutMin=[]  KbOutMax=[]  KtOutMin=[]  KtOutMax=[]  IntegratorOutMin=[]  IntegratorOutMax=[]  FilterOutMin=[]  FilterOutMax=[]  SumOutMin=[]  SumOutMax=[]  SumI1OutMin=[]  SumI1OutMax=[]  SumI2OutMin=[]  SumI2OutMax=[]  SumI3OutMin=[]  SumI3OutMax=[]  SumDOutMin=[]  SumDOutMax=[]  SaturationOutMin=[]  SaturationOutMax=[]  IntegratorContinuousStateAttributes=''  IntegratorStateMustResolveToSignalObject=off  IntegratorRTWStateStorageClass=Auto  FilterContinuousStateAttributes=''  FilterStateMustResolveToSignalObject=off  FilterRTWStateStorageClass=Auto  DifferentiatorICPrevScaledInput=0  DifferentiatorOutMin=[]  DifferentiatorOutMax=[]
  Rate Limiter : RateLimiter  RisingSlewLimit=10  FallingSlewLimit=-10
  Sum3 : Sum  Inputs=|+-  SampleTime=Ts
  t=Pitch_time_constant1 : powerlib_extras/Discrete  Control Blocks/Discrete 1st-Order Filter  FilterType=Lowpass  Tc=0.02  Ts=Ts  Initialize=on  Vac_Init=[0.8 -25 60]*0  Vdc_Init=0  PlotResponse=off  param1=[1 500 0.1]
  pitch : Outport
  wires:
  Sum3/1 -> Discrete PID Controller/1
  wg/1 -> Sum3/1
  Ref/1 -> Sum3/2
  Rate Limiter/1 -> "0-pitch_max "/1
  "0-pitch_max "/1 -> t=Pitch_time_constant1/1
  t=Pitch_time_constant1/1 -> pitch/1
  Discrete PID Controller/1 -> Rate Limiter/1

== system ieee_6_bus_modified/GE2.75 - 3/pitch angle controller/pitch angle controller ==
  wg : Inport
  Ref : Inport  Port=2
  "0-pitch_max " : Saturate  UpperLimit=27  LowerLimit=0  SampleTime=Ts
  Discrete PID Controller : simulink/Continuous/PID Controller  Controller=PI  TimeDomain=Discrete-time  SampleTime=Ts  IntegratorMethod=Forward Euler  FilterMethod=Forward Euler  Form=Parallel  UseFilter=on  ControllerParametersSource=internal  P=200  I=25  D=0  N=100  InitialConditionSource=internal  InitialConditionForIntegrator=0  InitialConditionForFilter=0  ExternalReset=none  ZeroCross=off  LimitOutput=on  UpperSaturationLimit=27  LowerSaturationLimit=0  LinearizeAsGain=off  AntiWindupMode=clamping  Kb=1  TrackingMode=off  Kt=1  PParamMin=[]  PParamMax=[]  IParamMin=[]  IParamMax=[]  DParamMin=[]  DParamMax=[]  NParamMin=[]  NParamMax=[]  KbParamMin=[]  KbParamMax=[]  KtParamMin=[]  KtParamMax=[]  POutMin=[]  POutMax=[]  IOutMin=[]  IOutMax=[]  DOutMin=[]  DOutMax=[]  NOutMin=[]  NOutMax=[]  KbOutMin=[]  KbOutMax=[]  KtOutMin=[]  KtOutMax=[]  IntegratorOutMin=[]  IntegratorOutMax=[]  FilterOutMin=[]  FilterOutMax=[]  SumOutMin=[]  SumOutMax=[]  SumI1OutMin=[]  SumI1OutMax=[]  SumI2OutMin=[]  SumI2OutMax=[]  SumI3OutMin=[]  SumI3OutMax=[]  SumDOutMin=[]  SumDOutMax=[]  SaturationOutMin=[]  SaturationOutMax=[]  IntegratorContinuousStateAttributes=''  IntegratorStateMustResolveToSignalObject=off  IntegratorRTWStateStorageClass=Auto  FilterContinuousStateAttributes=''  FilterStateMustResolveToSignalObject=off  FilterRTWStateStorageClass=Auto  DifferentiatorICPrevScaledInput=0  DifferentiatorOutMin=[]  DifferentiatorOutMax=[]
  Rate Limiter : RateLimiter  RisingSlewLimit=10  FallingSlewLimit=-10
  Sum3 : Sum  Inputs=|+-  SampleTime=Ts
  t=Pitch_time_constant1 : powerlib_extras/Discrete  Control Blocks/Discrete 1st-Order Filter  FilterType=Lowpass  Tc=0.02  Ts=Ts  Initialize=on  Vac_Init=[0.8 -25 60]*0  Vdc_Init=0  PlotResponse=off  param1=[1 500 0.1]
  pitch : Outport
  wires:
  Discrete PID Controller/1 -> Rate Limiter/1
  t=Pitch_time_constant1/1 -> pitch/1
  "0-pitch_max "/1 -> t=Pitch_time_constant1/1
  Rate Limiter/1 -> "0-pitch_max "/1
  Ref/1 -> Sum3/2
  wg/1 -> Sum3/1
  Sum3/1 -> Discrete PID Controller/1

== system ieee_6_bus_modified/GE2.75 - 4/pitch angle controller/pitch angle controller ==
  wg : Inport
  Ref : Inport  Port=2
  "0-pitch_max " : Saturate  UpperLimit=27  LowerLimit=0  SampleTime=Ts
  Discrete PID Controller : simulink/Continuous/PID Controller  Controller=PI  TimeDomain=Discrete-time  SampleTime=Ts  IntegratorMethod=Forward Euler  FilterMethod=Forward Euler  Form=Parallel  UseFilter=on  ControllerParametersSource=internal  P=200  I=25  D=0  N=100  InitialConditionSource=internal  InitialConditionForIntegrator=0  InitialConditionForFilter=0  ExternalReset=none  ZeroCross=off  LimitOutput=on  UpperSaturationLimit=27  LowerSaturationLimit=0  LinearizeAsGain=off  AntiWindupMode=clamping  Kb=1  TrackingMode=off  Kt=1  PParamMin=[]  PParamMax=[]  IParamMin=[]  IParamMax=[]  DParamMin=[]  DParamMax=[]  NParamMin=[]  NParamMax=[]  KbParamMin=[]  KbParamMax=[]  KtParamMin=[]  KtParamMax=[]  POutMin=[]  POutMax=[]  IOutMin=[]  IOutMax=[]  DOutMin=[]  DOutMax=[]  NOutMin=[]  NOutMax=[]  KbOutMin=[]  KbOutMax=[]  KtOutMin=[]  KtOutMax=[]  IntegratorOutMin=[]  IntegratorOutMax=[]  FilterOutMin=[]  FilterOutMax=[]  SumOutMin=[]  SumOutMax=[]  SumI1OutMin=[]  SumI1OutMax=[]  SumI2OutMin=[]  SumI2OutMax=[]  SumI3OutMin=[]  SumI3OutMax=[]  SumDOutMin=[]  SumDOutMax=[]  SaturationOutMin=[]  SaturationOutMax=[]  IntegratorContinuousStateAttributes=''  IntegratorStateMustResolveToSignalObject=off  IntegratorRTWStateStorageClass=Auto  FilterContinuousStateAttributes=''  FilterStateMustResolveToSignalObject=off  FilterRTWStateStorageClass=Auto  DifferentiatorICPrevScaledInput=0  DifferentiatorOutMin=[]  DifferentiatorOutMax=[]
  Rate Limiter : RateLimiter  RisingSlewLimit=10  FallingSlewLimit=-10
  Sum3 : Sum  Inputs=|+-  SampleTime=Ts
  t=Pitch_time_constant1 : powerlib_extras/Discrete  Control Blocks/Discrete 1st-Order Filter  FilterType=Lowpass  Tc=0.02  Ts=Ts  Initialize=on  Vac_Init=[0.8 -25 60]*0  Vdc_Init=0  PlotResponse=off  param1=[1 500 0.1]
  pitch : Outport
  wires:
  Sum3/1 -> Discrete PID Controller/1
  wg/1 -> Sum3/1
  Ref/1 -> Sum3/2
  Rate Limiter/1 -> "0-pitch_max "/1
  "0-pitch_max "/1 -> t=Pitch_time_constant1/1
  t=Pitch_time_constant1/1 -> pitch/1
  Discrete PID Controller/1 -> Rate Limiter/1

== matlab function ieee_6_bus_modified/GE2.75 - 1/MATLAB Function1 ==
  data: u input; B input; Cp output
function Cp = fcn(u,B)

c1 = 0.5176;
c2 = 116;
c3 = 0.4; 
c4 = 5;
c5 = 21;
c6 = 0.0068;

i =u;

li = 1/((1/(i+0.08*B))-(0.035/(B^3+1)));

Cp = c1*((c2/li-c3*B-c4)*exp(-c5/li))+c6*i;

end

== matlab function ieee_6_bus_modified/GE2.75 - 2/MATLAB Function1 ==
  data: u input; B input; Cp output
function Cp = fcn(u,B)

c1 = 0.5176;
c2 = 116;
c3 = 0.4; 
c4 = 5;
c5 = 21;
c6 = 0.0068;

i =u;

li = 1/((1/(i+0.08*B))-(0.035/(B^3+1)));

Cp = c1*((c2/li-c3*B-c4)*exp(-c5/li))+c6*i;

end

== matlab function ieee_6_bus_modified/GE2.75 - 3/MATLAB Function1 ==
  data: u input; B input; Cp output
function Cp = fcn(u,B)

c1 = 0.5176;
c2 = 116;
c3 = 0.4; 
c4 = 5;
c5 = 21;
c6 = 0.0068;

i =u;

li = 1/((1/(i+0.08*B))-(0.035/(B^3+1)));

Cp = c1*((c2/li-c3*B-c4)*exp(-c5/li))+c6*i;

end

== matlab function ieee_6_bus_modified/GE2.75 - 4/MATLAB Function1 ==
  data: u input; B input; Cp output
function Cp = fcn(u,B)

c1 = 0.5176;
c2 = 116;
c3 = 0.4; 
c4 = 5;
c5 = 21;
c6 = 0.0068;

i =u;

li = 1/((1/(i+0.08*B))-(0.035/(B^3+1)));

Cp = c1*((c2/li-c3*B-c4)*exp(-c5/li))+c6*i;

end
